simulink model "vehicle_dynamics_system"  (Simulink 7.7)
settings: Solver=ode3  StartTime=0.0  StopTime=10.0  FixedStep=T  RelTol=1e-3
PreLoadFcn:
  | init_parameters;
values from neighbouring files (symbols this model uses):
  CarBody =     [VehicleData_VectorCar.mat]
  Differential =     [VehicleData_VectorCar.mat]
  Engine =     [VehicleData_VectorCar.mat]
  Gearbox =     [VehicleData_VectorCar.mat]
  Ground =     [GroundData_Plane.mat]
  Suspension =     [VehicleData_VectorCar.mat]
  Wheel =     [VehicleData_VectorCar.mat]
libraries: vehicle_dynamics_lib x11, simulink x1
(part 1 of 3)
CloseFcn:
  | rtwprivate ssgencode ModelCloseRequest vehicle_dynamics_system
settings Model: Creator=vismso  LastModifiedBy=visjf
settings DataIOCC: SaveOutput=off  SignalLogging=off  SaveTime=off
settings OptimizationCC: InlineParams=on  UseIntDivNetSlope=on  SimCompilerOptimization=On
settings DebuggingCC: ArtificialAlgebraicLoopMsg=none  BusObjectLabelMismatch=error  RootOutportRequireBusObject=error  StrictBusMsg=Warning
settings SFSimCC: SimParseCustomCode=off
settings RTWCC: SystemTargetFile=cn.tlc  TemplateMakefile=cn_msdll.tmf  Description=Vector CANoe Real-Time Target DLL (Visual C/C++ Project Makefile)  ProcessScript=cn_make_rtw_hook
settings CodeAppCC: MaxIdLength=128  SimulinkBlockComments=off
settings STFCustomTargetCC: FunctionExecutionProfile=off  GeneratePreprocessorConditionals=Disable all  MatFileLogging=on  SystemTargetFile=cn.tlc
settings GRTTargetCC: ParMdlRefBuildCompliant=off  CompOptLevelCompliant=off  ExtModeMexFile=noextcomm  RTWCAPISignals=on  RTWCAPIParams=on
settings CustomProperty: DataType=string  Value=..\canoe

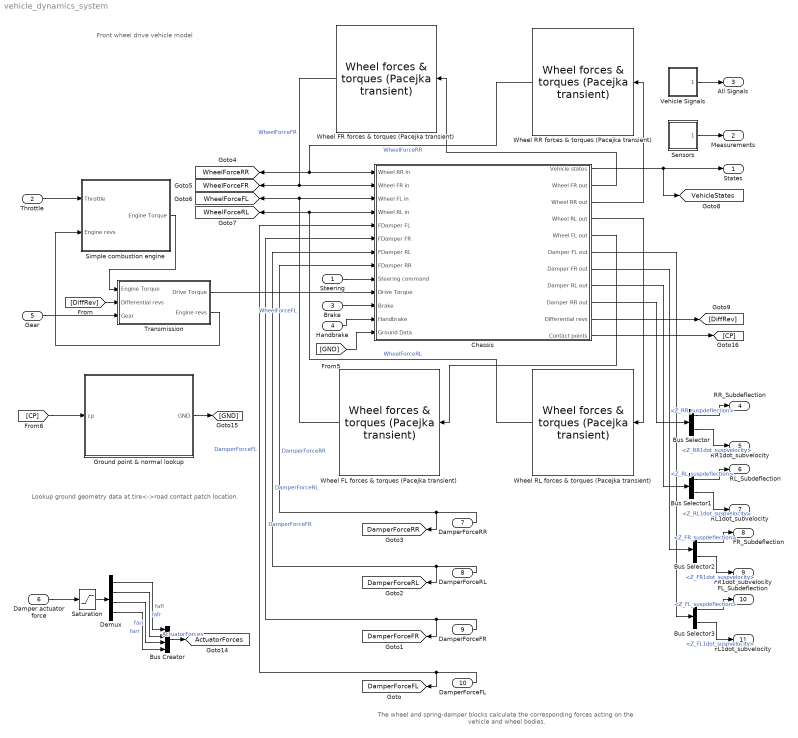
== system vehicle_dynamics_system ==
  note: Front wheel drive vehicle model
  note: The wheel and spring-damper blocks calculate
      | the corresponding forces acting on the vehicle and wheel bodies.
  note: Lookup ground geometry data
      | at tire<->road contact patch location.
  Steering : Inport
  Throttle : Inport  Port=2
  Brake : Inport  Port=3
  Handbrake : Inport  Port=4
  Gear : Inport  Port=5
  Damper actuator force : Inport  Port=6
  "DamperForceRR " : Inport  Port=7
  "DamperForceRL " : Inport  Port=8
  DamperForceFR : Inport  Port=9
  DamperForceFL : Inport  Port=10
  Bus Creator : BusCreator
  Bus Selector : BusSelector  OutputSignals=Z_RR_suspdeflection,Z_RR1dot_suspvelocity
  Bus Selector1 : BusSelector  OutputSignals=Z_RL_suspdeflection,Z_RL1dot_suspvelocity
  Bus Selector2 : BusSelector  OutputSignals=Z_FR_suspdeflection,Z_FR1dot_suspvelocity
  Bus Selector3 : BusSelector  OutputSignals=Z_FL_suspdeflection,Z_FL1dot_suspvelocity
  Chassis : Subsystem  mask{rFLWheelMountPoint=Suspension.MountPointFL, rFRWheelMountPoint=Suspension.MountPointFR, rRLWheelMountPoint=Suspension.MountPointRL, rRRWheelMountPoint=Suspension.MountPointRR, rFAirPointOfAttack=CarBody.FrontAirDragPointOfAttack, rRAirPointOfAttack=CarBody.RearAirDragPointOfAttack, g=9.81, c_ROLLBARF=Suspension.FrontRollbarStiffness, c_ROLLBARR=Suspension.RearRollbarStiffness, m_body=CarBody.Mass, m_wheel=Wheel.Mass, I_body=CarBody.InertiaTensor, I_wheel=Wheel.InertiaTensor}
      mask prompts: rFLWheelMountPoint "Mount point of front left damper in local body coordinates [m]"; rFRWheelMountPoint "Mount point of front right damper in local body coordinates [m]"; rRLWheelMountPoint "Mount point of rear left damper in local body coordinates [m]"; rRRWheelMountPoint "Mount point of rear right damper in local body coordinates [m]"; rFAirPointOfAttack "Front air drag force's point of attack in local body coordinates [m]"; rRAirPointOfAttack "Rear air drag force's point of attack in local body coordinates [m]"; g "Gravity in z-Direction [m/s^2]"; c_ROLLBARF "Front rollbar stiffness [N/m]"; c_ROLLBARR "Rear rollbar stiffness [N/m]"; m_body "Chassis mass [kg]"; m_wheel "Wheel mass [kg]"; I_body "Chassis inertia [kg m^2]"; I_wheel "Wheel inertia [kg m^2]"
      mask init:
      | inputs=find_system(gcb,'SearchDepth',1,'LookUnderMasks','on','BlockType','Inport');
      | outputs=find_system(gcb,'SearchDepth',1,'LookUnderMasks','on','BlockType','Outport');
      | 
      | for i = 1:length(inputs)
      |     s.(['inport' num2str(i)]) = str2num(get_param(inputs{i},'Port'));
      |     s.(['inname' num2str(i)]) = get_param(inputs{i},'Name');
      | end
      | 
      | for i = 1:length(outputs)
      |     s.(['outport' num2str(i)]) = str2num(get_param(outputs{i},'Port'));
      |     s.(['outname' num2str(i)]) = get_param(outputs{i},'Name');
      | end
      settings: MinAlgLoopOccurrences=on
      mask Display:
      | image(imread('chassis.jpg'))
      | 
      | color('white')
      | 
      | port_label('input',s.inport1,s.inname1)
      | port_label('input',s.inport2,s.inname2)
      | port_label('input',s.inport3,s.inname3)
      | port_label('input',s.inport4,s.inname4)
      | port_label('input',s.inport5,s.inname5)
      | port_label('input',s.inport6,s.inname6)
      | port_label('input',s.inport7,s.inname7)
      | port_label('input',s.inport8,s.inname8)
      | port_label('input',s.inport9,s.inname9)
      | port_label('input',s.inport10,s.inname10)
      | port_label('input',s.inport11,s.inname11)
      | port_label('input',s.inport12,s.inname12)
      | port_label('input',s.inport13,s.inname13)
      | 
      | port_label('output',s.outport1,s.outname1)
      | port_label('output',s.outport2,s.outname2)
      | port_label('output',s.outport3,s.outname3)
      | port_label('output',s.outport4,s.outname4)
      | port_label('output',s.outport5,s.outname5)
      | port_label('output',s.outport6,s.outname6)
      | port_label('output',s.outport7,s.outname7)
      | port_label('output',s.outport8,s.outname8)
      | port_label('output',s.outport9,s.outname9)
      | port_label('output',s.outport10,s.outname10)
      | port_label('output',s.outport11,s.outname11)
  Demux : Demux
  Ground point & normal lookup : Subsystem  mask{X=Ground.X, Y=Ground.Y, Z=Ground.Z, Nx=Ground.NormalX, Ny=Ground.NormalY, Nz=Ground.NormalZ}
      mask prompts: X "Ground X grid"; Y "Ground Y grid"; Z "Ground Z values"; Nx "Ground normals (x component)"; Ny "Ground normals (y component)"; Nz "Ground normals (x component)"
      mask Display:
      | image(imread('asphalt.jpg'))
      | color('white')
      | port_label('output',1,'Ground Data')
      | port_label('input',1,'Contact Point')
  Saturation : Saturate  UpperLimit=6e3  LowerLimit=-6e3
  Sensors : Subsystem
      mask init:
      | x=-1:0.05:1;
      | y=sqrt(1-x.^2);
      mask Display:
      | plot((x+1)/2,y/2+.5)
      | plot([0 1/sqrt(2)]/2.5+.5,[0,1/sqrt(2)]/2.5+.5)
  Simple combustion engine : Subsystem
      mask init: same as vehicle_dynamics_system/Chassis
      mask Display:
      | image(imread('engine.jpg'))
      | 
      | color('white')
      | 
      | port_label('input',s.inport1,s.inname1)
      | port_label('input',s.inport2,s.inname2)
      | 
      | port_label('output',s.outport1,s.outname1)
  Transmission : Subsystem  mask(Transmission Block){nGears=Gearbox.Ratios}
      mask prompts: nGears "Gear ratios (1st entry is reverse gear and should be negative)"
      mask help:
      | This block represents the transmission of a vehicle. Set the gear ratios in
      | the input field. Any number of gears greater than zero ist allowed. The
      | first entry usually represents the ratio of the reverse gear and should
      | therefor be negative.
      |
      | Example: [-4;3.827;2.793;2.039;1.488;1.086;0.793]
      | This defines 7 gears.
      mask Help:
      | This block represents the transmission of a vehicle. Set the gear ratios in
      | the input field. Any number of gears greater than zero ist allowed. The
      | first entry usually represents the ratio of the reverse gear and should
      | therefor be negative.
      | 
      | Example: [-4;3.827;2.793;2.039;1.488;1.086;0.793]
      | 
      | This defines 7 gears:
      | R:  -4
      | 1:  3.827
      | 2:  2.793
      | 3:  2.039
      | 4:  1.488
      | 5:  1.086
      | 6:  0.793
      | 
      | With the GEAR input you can select the used gear. A zero at the input means
      | using the first defined ratio, in this case the reverse gear.
      | 
      | The ENGINE REVS output calculates the engine's revs in rad/s according to
      | the DIFFERENTIAL REVS input: omega_engine = GearRatio * omega_diff
      | 
      | The DRIVE TORQUE output calculates the torque applied to the diff with
      | respect to the ENGINE TORQUE input: M_diff = GearRatio * M_engine
  Vehicle Signals : Subsystem
      mask init:
      | x=-1:0.05:1;
      | y=sqrt(1-x.^2);
      mask Display:
      | plot((x+1)/2,y/2+.5)
      | plot([0 1/sqrt(2)]/2.5+.5,[0,1/sqrt(2)]/2.5+.5)
  Wheel FL forces & torques (Pacejka transient) : vehicle_dynamics_lib/Force elements/Wheel forces & torques (Pacejka transient)  SystemSampleTime=-1  c=Wheel.TireStiffness  d=Wheel.TireDamping  r0=Wheel.UnloadedRadius  a=Wheel.PacejkaLateral  b=Wheel.PacejkaLongitudinal  Lx=Wheel.RelaxationLongitudinal  Ly=Wheel.RelaxationLateral  Vlow=Wheel.SlipDampingLowerSpeedLimit
  Wheel FR forces & torques (Pacejka transient) : vehicle_dynamics_lib/Force elements/Wheel forces & torques (Pacejka transient)  SystemSampleTime=-1  c=Wheel.TireStiffness  d=Wheel.TireDamping  r0=Wheel.UnloadedRadius  a=Wheel.PacejkaLateral  b=Wheel.PacejkaLongitudinal  Lx=Wheel.RelaxationLongitudinal  Ly=Wheel.RelaxationLateral  Vlow=Wheel.SlipDampingLowerSpeedLimit
  Wheel RL forces & torques (Pacejka transient) : vehicle_dynamics_lib/Force elements/Wheel forces & torques (Pacejka transient)  SystemSampleTime=-1  c=Wheel.TireStiffness  d=Wheel.TireDamping  r0=Wheel.UnloadedRadius  a=Wheel.PacejkaLateral  b=Wheel.PacejkaLongitudinal  Lx=Wheel.RelaxationLongitudinal  Ly=Wheel.RelaxationLateral  Vlow=Wheel.SlipDampingLowerSpeedLimit
  Wheel RR forces & torques (Pacejka transient) : vehicle_dynamics_lib/Force elements/Wheel forces & torques (Pacejka transient)  SystemSampleTime=-1  c=Wheel.TireStiffness  d=Wheel.TireDamping  r0=Wheel.UnloadedRadius  a=Wheel.PacejkaLateral  b=Wheel.PacejkaLongitudinal  Lx=Wheel.RelaxationLongitudinal  Ly=Wheel.RelaxationLateral  Vlow=Wheel.SlipDampingLowerSpeedLimit
  States : Outport  OutDataTypeStr=Bus: Bus_Vehicle
  Measurements : Outport  Port=2  OutDataTypeStr=Bus: Bus_Measurements
  All Signals : Outport  Port=3  OutDataTypeStr=Bus: Bus_VehicleSignals
  RR_Subdeflection : Outport  Port=4
  RR1dot_subvelocity : Outport  Port=5
  RL_Subdeflection : Outport  Port=6
  RL1dot_subvelocity : Outport  Port=7
  FR_Subdeflection : Outport  Port=8
  FR1dot_subvelocity : Outport  Port=9
  FL_Subdeflection : Outport  Port=10
  FL1dot_subvelocity : Outport  Port=11
  tag scope: ActuatorForces=global, DamperForceFL=global, DamperForceFR=global, DamperForceRL=global, DamperForceRR=global, VehicleStates=global, WheelForceFL=global, WheelForceFR=global, WheelForceRL=global, WheelForceRR=global
  wires:
  Wheel FL forces & torques (Pacejka transient)/1 -> Chassis/3(Wheel FL in), [WheelForceFL]  "WheelForceFL"
  Chassis/5(Wheel FL out) -> Wheel FL forces & torques (Pacejka transient)/1
  Chassis/2(Wheel FR out) -> Wheel FR forces & torques (Pacejka transient)/1
  Wheel FR forces & torques (Pacejka transient)/1 -> Chassis/2(Wheel FR in), [WheelForceFR]  "WheelForceFR"
  Chassis/4(Wheel RL out) -> Wheel RL forces & torques (Pacejka transient)/1
  Chassis/3(Wheel RR out) -> Wheel RR forces & torques (Pacejka transient)/1
  Wheel RR forces & torques (Pacejka transient)/1 -> Chassis/1(Wheel RR in), [WheelForceRR]  "WheelForceRR"
  Wheel RL forces & torques (Pacejka transient)/1 -> Chassis/4(Wheel RL in), [WheelForceRL]  "WheelForceRL"
  Chassis/6(Damper FL out) -> Bus Selector3/1
  Chassis/7(Damper FR out) -> Bus Selector2/1
  Chassis/8(Damper RL out) -> Bus Selector1/1
  Chassis/9(Damper RR out) -> Bus Selector/1
  DamperForceFL/1 -> [DamperForceFL], Chassis/5(FDamper FL)  "DamperForceFL"
  DamperForceFR/1 -> [DamperForceFR], Chassis/6(FDamper FR)  "DamperForceFR"
  "DamperForceRL "/1 -> [DamperForceRL], Chassis/7(FDamper RL)  "DamperForceRL"
  "DamperForceRR "/1 -> [DamperForceRR], Chassis/8(FDamper RR)  "DamperForceRR"
  Chassis/1(Vehicle states) -> States/1, [VehicleStates]
  Steering/1 -> Chassis/9(Steering command)
  Throttle/1 -> Simple combustion engine/1(Throttle)
  Transmission/1(Drive Torque) -> Chassis/10(Drive Torque)
  Simple combustion engine/1(Engine Torque) -> Transmission/1(Engine Torque)
  Transmission/2(Engine revs) -> Simple combustion engine/2(Engine revs)
  Gear/1 -> Transmission/3(Gear)
  Brake/1 -> Chassis/11(Brake)
  Sensors/1(Measurements) -> Measurements/1
  Damper actuator force/1 -> Saturation/1
  [DiffRev] -> Transmission/2(Differential revs)
  Chassis/10(Differential revs) -> [DiffRev]
  Demux/1 -> Bus Creator/1  "fafl"
  Demux/2 -> Bus Creator/2  "fafr"
  Demux/3 -> Bus Creator/3  "farl"
  Demux/4 -> Bus Creator/4  "farr"
  Handbrake/1 -> Chassis/12(Handbrake)
  [GND] -> Chassis/13(Ground Data)
  Ground point & normal lookup/1(GND) -> [GND]
  [CP] -> Ground point & normal lookup/1(cp)
  Chassis/11(Contact points) -> [CP]
  Saturation/1 -> Demux/1
  Bus Creator/1 -> [ActuatorForces]  "ActuatorForces"
  Vehicle Signals/1(Vehicle Signals) -> All Signals/1
  Bus Selector/1 -> RR_Subdeflection/1  "<Z_RR_suspdeflection>"
  Bus Selector/2 -> RR1dot_subvelocity/1  "<Z_RR1dot_suspvelocity>"
  Bus Selector1/1 -> RL_Subdeflection/1  "<Z_RL_suspdeflection>"
  Bus Selector1/2 -> RL1dot_subvelocity/1  "<Z_RL1dot_suspvelocity>"
  Bus Selector2/1 -> FR_Subdeflection/1  "<Z_FR_suspdeflection>"
  Bus Selector2/2 -> FR1dot_subvelocity/1  "<Z_FR1dot_suspvelocity>"
  Bus Selector3/1 -> FL_Subdeflection/1  "<Z_FL_suspdeflection>"
  Bus Selector3/2 -> FL1dot_subvelocity/1  "<Z_FL1dot_suspvelocity>"

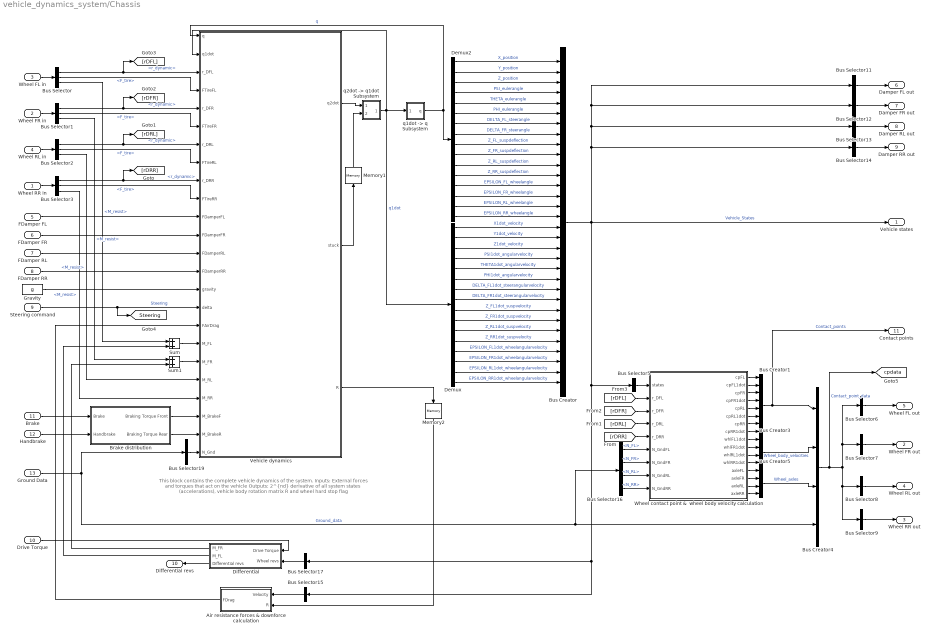
== system vehicle_dynamics_system/Chassis ==
  note: This block contains the complete vehicle dynamics of the system.
      | Inputs: External forces and torques that act on the vehicle
      | Outputs: 2^{nd} derivative of all system states (accelerations), vehicle body rotation matrix R and wheel hard stop flag
  Wheel RR in : Inport
  Wheel FR in : Inport  Port=2
  Wheel FL in : Inport  Port=3
  Wheel RL in : Inport  Port=4
  FDamper FL : Inport  Port=5
  FDamper FR : Inport  Port=6
  FDamper RL : Inport  Port=7
  FDamper RR : Inport  Port=8
  Steering command : Inport  Port=9
  Drive Torque : Inport  Port=10
  Brake : Inport  Port=11
  Handbrake : Inport  Port=12
  Ground Data : Inport  Port=13
  Air resistance forces & downforce calculation : Subsystem  mask{Cw=0.37, Ksfront=0.12, Ksrear=0.16, rho=1.2, A=1.85}
      mask prompts: Cw "Drag coefficient"; Ksfront "Front wing coefficient"; Ksrear "Rear wing coefficient"; rho "Air density [kg/m^3]"; A "Frontal area [m^2]"
  Brake distribution : Subsystem  mask{nBrakeF=0.8, M_Max=4000, M_HBMax=1000}
      mask prompts: nBrakeF "Braking force distribution to front wheels"; M_Max "Maximum braking torque [Nm]"; M_HBMax "Maximum handbrake torque [Nm]"
      mask CallbackString:
      | if or(str2num(get_param(gcb, 'nBrakeF'))<0, str2num(get_param(gcb, 'nBrakeF'))>1)
      | 	error('Brake distribution must be between zero and one.')
      | end||
  Bus Creator : BusCreator  Inputs=32
  Bus Creator1 : BusCreator  Inputs=8
  Bus Creator3 : BusCreator
  Bus Creator4 : BusCreator
  Bus Creator5 : BusCreator
  Bus Selector{,1..3} (4 alike) : BusSelector  OutputSignals=r_dynamic,F_tire,M_resist
  Bus Selector11 : BusSelector  OutputSignals=Z_FL_suspdeflection,Z_FL1dot_suspvelocity  OutputAsBus=on
  Bus Selector12 : BusSelector  OutputSignals=Z_FR_suspdeflection,Z_FR1dot_suspvelocity  OutputAsBus=on
  Bus Selector13 : BusSelector  OutputSignals=Z_RL_suspdeflection,Z_RL1dot_suspvelocity  OutputAsBus=on
  Bus Selector14 : BusSelector  OutputSignals=Z_RR_suspdeflection,Z_RR1dot_suspvelocity  OutputAsBus=on
  Bus Selector15 : BusSelector  OutputSignals=X1dot_velocity,Y1dot_velocity,Z1dot_velocity  OutputAsBus=on
  Bus Selector16 : BusSelector  OutputSignals=GND_FL.N_FL,GND_FR.N_FR,GND_RL.N_RL,GND_RR.N_RR
  Bus Selector17 : BusSelector  OutputSignals=EPSILON_FL1dot_wheelangularvelocity,EPSILON_FR1dot_wheelangularvelocity  OutputAsBus=on
  Bus Selector19 : BusSelector  OutputSignals=GND_FL.N_FL,GND_FR.N_FR,GND_RL.N_RL,GND_RR.N_RR  OutputAsBus=on
  Bus Selector5 : BusSelector  OutputSignals=X_position,Y_position,Z_position,PSI_eulerangle,THETA_eulerangle,PHI_eulerangle,DELTA_FL_steerangle,DELTA_FR_steerangle,Z_FL_suspdeflection,Z_FR_suspdeflection,Z_RL_suspdeflection,Z_RR_suspdeflection,X1dot_velocity,Y1dot_velocity,Z1dot_velocity,PSI1dot_angularvelocity,THETA1dot_angularvelocity,PHI1dot_angularvelocity,Z_FL1dot_suspvelocity,Z_FR1dot_suspvelocity,Z_RL1dot_suspvelocity,Z_RR1dot_suspvelocity,EPSILON_FL1dot_wheelangularvelocity,EPSILON_FR1dot_wheelangularvelocity,EPSILON_RL1dot_wheelangularvelocity,EPSILON_RR1dot_wheelangularvelocity  OutputAsBus=on
  Bus Selector6 : BusSelector  OutputSignals=Wheel_axles.axleFL,Contact_points.cpFL,Contact_points.cpFL1dot,Wheel_body_velocities.whlFL1dot,Ground_data.GND_FL  OutputAsBus=on
  Bus Selector7 : BusSelector  OutputSignals=Wheel_axles.axleFR,Contact_points.cpFR,Contact_points.cpFR1dot,Wheel_body_velocities.whlFR1dot,Ground_data.GND_FR  OutputAsBus=on
  Bus Selector8 : BusSelector  OutputSignals=Wheel_axles.axleRL,Contact_points.cpRL,Contact_points.cpRL1dot,Wheel_body_velocities.whlRL1dot,Ground_data.GND_RL  OutputAsBus=on
  Bus Selector9 : BusSelector  OutputSignals=Wheel_axles.axleRR,Contact_points.cpRR,Contact_points.cpRR1dot,Wheel_body_velocities.whlRR1dot,Ground_data.GND_RR  OutputAsBus=on
  Demux : Demux  Outputs=16
  Demux2 : Demux  Outputs=16
  Differential : Subsystem  mask{nd=Differential.Ratio}
      mask prompts: nd "Differential ratio"
  Gravity : Constant  Value=g
  Memory1 : Memory
  Memory2 : Memory
  Sum : Sum
  Sum1 : Sum
  Vehicle dynamics : Stateflow chart  RequirementInfo={} %GIDa_b7f5b320_cde6_4ae1_9d3b_3c9937b9ba5b  TreatAsAtomicUnit=on
  Wheel contact point &  wheel body velocity calculation : Stateflow chart  TreatAsAtomicUnit=on
      settings: MinAlgLoopOccurrences=on
  "q1dot -> q Subsystem" : Subsystem
      mask Display:
      | droots([],[0],1)
      | plot([1 1.5 1.7 2],[0 0 2 2])
      | plot(6,6)
  "q2dot -> q1dot Subsystem" : Subsystem
      mask Display:
      | droots([],[0],1)
      | plot([1 1 2 2],[0 2 2 0])
      | plot([2 2.4 2.4],[2 2 0])
      | plot(7,7)
  Vehicle states : Outport
  Wheel FR out : Outport  Port=2
  Wheel RR out : Outport  Port=3
  Wheel RL out : Outport  Port=4
  Wheel FL out : Outport  Port=5
  Damper FL out : Outport  Port=6
  Damper FR out : Outport  Port=7
  Damper RL out : Outport  Port=8
  Damper RR out : Outport  Port=9
  Differential revs : Outport  Port=10
  Contact points : Outport  Port=11
  tag scope: Steering=global, cpdata=global
  wires:
  Vehicle dynamics/1(q2dot) -> "q2dot -> q1dot Subsystem"/1(q2dot)
  "q1dot -> q Subsystem"/1(q) -> Demux2/1, Vehicle dynamics/1(q)  "q"
  Wheel FL in/1 -> Bus Selector/1
  Bus Selector/1 -> Vehicle dynamics/3(r_DFL), [rDFL]  "<r_dynamic>"
  Wheel FR in/1 -> Bus Selector1/1
  Wheel RL in/1 -> Bus Selector2/1
  Wheel RR in/1 -> Bus Selector3/1
  Bus Selector1/1 -> Vehicle dynamics/5(r_DFR), [rDFR]  "<r_dynamic>"
  Bus Selector1/2 -> Vehicle dynamics/6(FTireFR)  "<F_tire>"
  Bus Selector2/1 -> Vehicle dynamics/7(r_DRL), [rDRL]  "<r_dynamic>"
  Bus Selector2/2 -> Vehicle dynamics/8(FTireRL)  "<F_tire>"
  Bus Selector3/1 -> Vehicle dynamics/9(r_DRR), [rDRR]  "<r_dynamic>"
  Bus Selector3/2 -> Vehicle dynamics/10(FTireRR)  "<F_tire>"
  FDamper FL/1 -> Vehicle dynamics/11(FDamperFL)
  FDamper FR/1 -> Vehicle dynamics/12(FDamperFR)
  FDamper RL/1 -> Vehicle dynamics/13(FDamperRL)
  FDamper RR/1 -> Vehicle dynamics/14(FDamperRR)
  Gravity/1 -> Vehicle dynamics/15(gravity)
  Bus Creator/1 -> Vehicle states/1, Bus Selector11/1, Bus Selector12/1, Bus Selector13/1, Bus Selector14/1, Bus Selector5/1, Bus Selector15/1, Bus Selector17/1  "Vehicle_States"
  Demux/1 -> Bus Creator/17  "X1dot_velocity"
  Demux/2 -> Bus Creator/18  "Y1dot_velocity"
  Demux/3 -> Bus Creator/19  "Z1dot_velocity"
  Demux/4 -> Bus Creator/20  "PSI1dot_angularvelocity"
  Demux/5 -> Bus Creator/21  "THETA1dot_angularvelocity"
  Demux/6 -> Bus Creator/22  "PHI1dot_angularvelocity"
  Demux/7 -> Bus Creator/23  "DELTA_FL1dot_steerangularvelocity"
  Demux/8 -> Bus Creator/24  "DELTA_FR1dot_steerangularvelocity"
  Demux/9 -> Bus Creator/25  "Z_FL1dot_suspvelocity"
  Demux/10 -> Bus Creator/26  "Z_FR1dot_suspvelocity"
  Demux/11 -> Bus Creator/27  "Z_RL1dot_suspvelocity"
  Demux/12 -> Bus Creator/28  "Z_RR1dot_suspvelocity"
  Demux/13 -> Bus Creator/29  "EPSILON_FL1dot_wheelangularvelocity"
  Demux/14 -> Bus Creator/30  "EPSILON_FR1dot_wheelangularvelocity"
  Demux/15 -> Bus Creator/31  "EPSILON_RL1dot_wheelangularvelocity"
  Demux/16 -> Bus Creator/32  "EPSILON_RR1dot_wheelangularvelocity"
  Demux2/1 -> Bus Creator/1  "X_position"
  Demux2/2 -> Bus Creator/2  "Y_position"
  Demux2/3 -> Bus Creator/3  "Z_position"
  Demux2/4 -> Bus Creator/4  "PSI_eulerangle"
  Demux2/5 -> Bus Creator/5  "THETA_eulerangle"
  Demux2/6 -> Bus Creator/6  "PHI_eulerangle"
  Demux2/9 -> Bus Creator/9  "Z_FL_suspdeflection"
  Demux2/10 -> Bus Creator/10  "Z_FR_suspdeflection"
  Demux2/11 -> Bus Creator/11  "Z_RL_suspdeflection"
  Demux2/12 -> Bus Creator/12  "Z_RR_suspdeflection"
  Demux2/13 -> Bus Creator/13  "EPSILON_FL_wheelangle"
  Demux2/14 -> Bus Creator/14  "EPSILON_FR_wheelangle"
  Demux2/15 -> Bus Creator/15  "EPSILON_RL_wheelangle"
  Demux2/16 -> Bus Creator/16  "EPSILON_RR_wheelangle"
  Steering command/1 -> Vehicle dynamics/16(delta), [Steering]  "Steering"
  Demux2/7 -> Bus Creator/7  "DELTA_FL_steerangle"
  Demux2/8 -> Bus Creator/8  "DELTA_FR_steerangle"
  Bus Creator1/1 -> Bus Creator4/1, Contact points/1  "Contact_points"
  Wheel contact point &  wheel body velocity calculation/1(cpFL) -> Bus Creator1/1
  Wheel contact point &  wheel body velocity calculation/2(cpFL1dot) -> Bus Creator1/2
  Wheel contact point &  wheel body velocity calculation/3(cpFR) -> Bus Creator1/3
  Wheel contact point &  wheel body velocity calculation/4(cpFR1dot) -> Bus Creator1/4
  Wheel contact point &  wheel body velocity calculation/5(cpRL) -> Bus Creator1/5
  Wheel contact point &  wheel body velocity calculation/6(cpRL1dot) -> Bus Creator1/6
  Wheel contact point &  wheel body velocity calculation/7(cpRR) -> Bus Creator1/7
  Wheel contact point &  wheel body velocity calculation/8(cpRR1dot) -> Bus Creator1/8
  Wheel contact point &  wheel body velocity calculation/9(whlFL1dot) -> Bus Creator3/1
  Wheel contact point &  wheel body velocity calculation/10(whlFR1dot) -> Bus Creator3/2
  Wheel contact point &  wheel body velocity calculation/11(whlRL1dot) -> Bus Creator3/3
  Wheel contact point &  wheel body velocity calculation/12(whlRR1dot) -> Bus Creator3/4
  Bus Selector5/1 -> Wheel contact point &  wheel body velocity calculation/1(states)
  Bus Creator4/1 -> Bus Selector7/1, Bus Selector6/1, Bus Selector9/1, Bus Selector8/1, [cpdata]  "Contact_point_data"
  Bus Selector6/1 -> Wheel FL out/1
  Bus Selector7/1 -> Wheel FR out/1
  Bus Selector8/1 -> Wheel RL out/1
  Bus Selector9/1 -> Wheel RR out/1
  Bus Selector11/1 -> Damper FL out/1
  Bus Selector12/1 -> Damper FR out/1
  Bus Selector13/1 -> Damper RL out/1
  Bus Selector14/1 -> Damper RR out/1
  Bus Selector15/1 -> Air resistance forces & downforce calculation/1(Velocity)
  Air resistance forces & downforce calculation/1(FDrag) -> Vehicle dynamics/17(FAirDrag)
  Sum/1 -> Vehicle dynamics/18(M_FL)
  Sum1/1 -> Vehicle dynamics/19(M_FR)
  Bus Selector/3 -> Sum/1  "<M_resist>"
  Bus Selector1/3 -> Sum1/1  "<M_resist>"
  Bus Selector2/3 -> Vehicle dynamics/20(M_RL)  "<M_resist>"
  Bus Selector3/3 -> Vehicle dynamics/21(M_RR)  "<M_resist>"
  Bus Creator5/1 -> Bus Creator4/3  "Wheel_axles"
  Wheel contact point &  wheel body velocity calculation/13(axleFL) -> Bus Creator5/1
  Wheel contact point &  wheel body velocity calculation/14(axleFR) -> Bus Creator5/2
  Wheel contact point &  wheel body velocity calculation/15(axleRL) -> Bus Creator5/3
  Wheel contact point &  wheel body velocity calculation/16(axleRR) -> Bus Creator5/4
  Bus Creator3/1 -> Bus Creator4/2  "Wheel_body_velocities"
  Drive Torque/1 -> Differential/1(Drive Torque)
  Differential/2(M_FL) -> Sum/2
  Differential/1(M_FR) -> Sum1/2
  Bus Selector17/1 -> Differential/2(Wheel revs)
  Differential/3(Differential revs) -> Differential revs/1
  [rDFL] -> Wheel contact point &  wheel body velocity calculation/2(r_DFL)
  [rDFR] -> Wheel contact point &  wheel body velocity calculation/3(r_DFR)
  [rDRL] -> Wheel contact point &  wheel body velocity calculation/4(r_DRL)
  [rDRR] -> Wheel contact point &  wheel body velocity calculation/5(r_DRR)
  Brake/1 -> Brake distribution/1(Brake)
  Brake distribution/1(Braking Torque Front) -> Vehicle dynamics/22(M_BrakeF)
  Brake distribution/2(Braking Torque Rear) -> Vehicle dynamics/23(M_BrakeR)
  Vehicle dynamics/3(R) -> Memory2/1
  "q2dot -> q1dot Subsystem"/1(q1dot) -> Demux/1, Vehicle dynamics/2(q1dot), "q1dot -> q Subsystem"/1(q1dot)  "q1dot"
  Vehicle dynamics/2(stuck) -> Memory1/1
  Memory2/1 -> Air resistance forces & downforce calculation/2(R)
  Memory1/1 -> "q2dot -> q1dot Subsystem"/2(Wheel revs reset)
  Ground Data/1 -> Bus Selector19/1, Bus Selector16/1, Bus Creator4/4  "Ground_data"
  Bus Selector16/1 -> Wheel contact point &  wheel body velocity calculation/6(N_GndFL)  "<N_FL>"
  Bus Selector16/2 -> Wheel contact point &  wheel body velocity calculation/7(N_GndFR)  "<N_FR>"
  Bus Selector16/3 -> Wheel contact point &  wheel body velocity calculation/8(N_GndRL)  "<N_RL>"
  Bus Selector16/4 -> Wheel contact point &  wheel body velocity calculation/9(N_GndRR)  "<N_RR>"
  Bus Selector19/1 -> Vehicle dynamics/24(N_Gnd)
  Handbrake/1 -> Brake distribution/2(Handbrake)
  Bus Selector/2 -> Vehicle dynamics/4(FTireFL)  "<F_tire>"

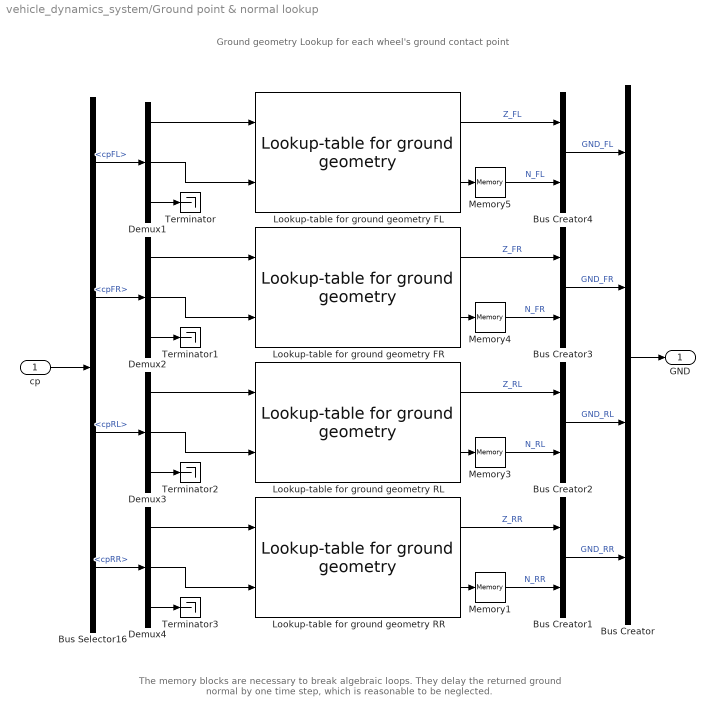
== system vehicle_dynamics_system/Ground point & normal lookup ==
  note: The memory blocks are necessary to break algebraic loops.
      | They delay the returned ground normal by one time step, which
      | is reasonable to be neglected.
  note: Ground geometry Lookup for each wheel's ground contact point
  cp : Inport
  Bus Creator : BusCreator
  Bus Creator{1..4} (4 alike) : BusCreator  Inputs=2
  Bus Selector16 : BusSelector  OutputSignals=cpFL,cpFR,cpRL,cpRR
  Demux{1..4} (4 alike) : Demux  Outputs=3
  Lookup-table for ground geometry FL : vehicle_dynamics_lib/Helper blocks/Lookup-table for ground geometry  SystemSampleTime=-1
  Lookup-table for ground geometry FR : vehicle_dynamics_lib/Helper blocks/Lookup-table for ground geometry  SystemSampleTime=-1
  Lookup-table for ground geometry RL : vehicle_dynamics_lib/Helper blocks/Lookup-table for ground geometry  SystemSampleTime=-1
  Lookup-table for ground geometry RR : vehicle_dynamics_lib/Helper blocks/Lookup-table for ground geometry  SystemSampleTime=-1
  Memory{1,3..5} (4 alike) : Memory  X0=[0;0;1]
  Terminator{,1..3} (4 alike) : Terminator
  GND : Outport
  wires:
  Bus Selector16/1 -> Demux1/1  "<cpFL>"
  cp/1 -> Bus Selector16/1
  Bus Selector16/2 -> Demux2/1  "<cpFR>"
  Bus Selector16/3 -> Demux3/1  "<cpRL>"
  Bus Selector16/4 -> Demux4/1  "<cpRR>"
  Demux1/1 -> Lookup-table for ground geometry FL/1
  Demux1/2 -> Lookup-table for ground geometry FL/2
  Demux2/1 -> Lookup-table for ground geometry FR/1
  Demux2/2 -> Lookup-table for ground geometry FR/2
  Demux3/1 -> Lookup-table for ground geometry RL/1
  Demux3/2 -> Lookup-table for ground geometry RL/2
  Demux4/1 -> Lookup-table for ground geometry RR/1
  Demux4/2 -> Lookup-table for ground geometry RR/2
  Demux1/3 -> Terminator/1
  Demux2/3 -> Terminator1/1
  Demux3/3 -> Terminator2/1
  Demux4/3 -> Terminator3/1
  Lookup-table for ground geometry FL/1 -> Bus Creator4/1  "Z_FL"
  Lookup-table for ground geometry FL/2 -> Memory5/1
  Lookup-table for ground geometry FR/1 -> Bus Creator3/1  "Z_FR"
  Lookup-table for ground geometry FR/2 -> Memory4/1
  Lookup-table for ground geometry RL/1 -> Bus Creator2/1  "Z_RL"
  Lookup-table for ground geometry RL/2 -> Memory3/1
  Lookup-table for ground geometry RR/1 -> Bus Creator1/1  "Z_RR"
  Lookup-table for ground geometry RR/2 -> Memory1/1
  Bus Creator4/1 -> Bus Creator/1  "GND_FL"
  Bus Creator3/1 -> Bus Creator/2  "GND_FR"
  Bus Creator2/1 -> Bus Creator/3  "GND_RL"
  Bus Creator1/1 -> Bus Creator/4  "GND_RR"
  Bus Creator/1 -> GND/1
  Memory1/1 -> Bus Creator1/2  "N_RR"
  Memory3/1 -> Bus Creator2/2  "N_RL"
  Memory4/1 -> Bus Creator3/2  "N_FR"
  Memory5/1 -> Bus Creator4/2  "N_FL"

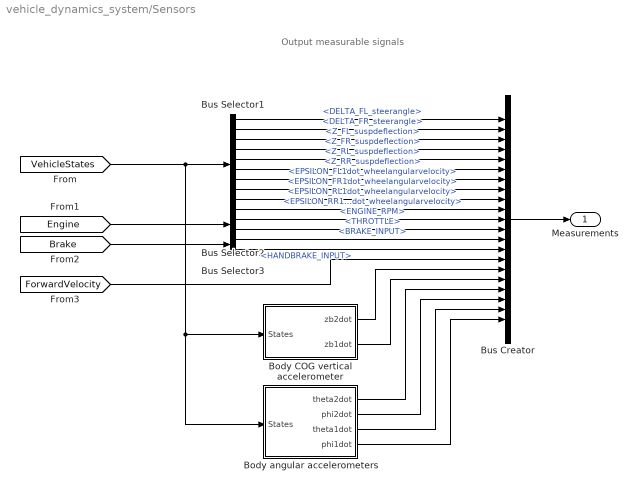
== system vehicle_dynamics_system/Sensors ==
  note: Output measurable signals
  Body COG vertical accelerometer : Subsystem
  Body angular accelerometers : Subsystem
  Bus Creator : BusCreator  Inputs=21
  Bus Selector1 : BusSelector  OutputSignals=DELTA_FL_steerangle,DELTA_FR_steerangle,Z_FL_suspdeflection,Z_FR_suspdeflection,Z_RL_suspdeflection,Z_RR_suspdeflection,EPSILON_FL1dot_wheelangularvelocity,EPSILON_FR1dot_wheelangularvelocity,EPSILON_RL1dot_wheelangularvelocity,EPSILON_RR1dot_wheelangularvelocity
  Bus Selector2 : BusSelector  OutputSignals=ENGINE_RPM,THROTTLE
  Bus Selector3 : BusSelector  OutputSignals=BRAKE_INPUT,HANDBRAKE_INPUT
  Measurements : Outport  OutDataTypeStr=Bus: Bus_Measurements
  wires:
  [VehicleStates] -> Body COG vertical accelerometer/1(States), Body angular accelerometers/1(States), Bus Selector1/1
  [Engine] -> Bus Selector2/1
  [Brake] -> Bus Selector3/1
  Bus Creator/1 -> Measurements/1
  Bus Selector1/1 -> Bus Creator/1  "<DELTA_FL_steerangle>"
  Bus Selector1/2 -> Bus Creator/2  "<DELTA_FR_steerangle>"
  Bus Selector1/3 -> Bus Creator/3  "<Z_FL_suspdeflection>"
  Bus Selector1/4 -> Bus Creator/4  "<Z_FR_suspdeflection>"
  Bus Selector1/5 -> Bus Creator/5  "<Z_RL_suspdeflection>"
  Bus Selector1/6 -> Bus Creator/6  "<Z_RR_suspdeflection>"
  Bus Selector1/7 -> Bus Creator/7  "<EPSILON_FL1dot_wheelangularvelocity>"
  Bus Selector1/8 -> Bus Creator/8  "<EPSILON_FR1dot_wheelangularvelocity>"
  Bus Selector1/9 -> Bus Creator/9  "<EPSILON_RL1dot_wheelangularvelocity>"
  Bus Selector1/10 -> Bus Creator/10  "<EPSILON_RR1dot_wheelangularvelocity>"
  Bus Selector2/1 -> Bus Creator/11  "<ENGINE_RPM>"
  Bus Selector2/2 -> Bus Creator/12  "<THROTTLE>"
  Bus Selector3/1 -> Bus Creator/13  "<BRAKE_INPUT>"
  Bus Selector3/2 -> Bus Creator/14  "<HANDBRAKE_INPUT>"
  [ForwardVelocity] -> Bus Creator/15
  Body COG vertical accelerometer/1(zb2dot) -> Bus Creator/16
  Body COG vertical accelerometer/2(zb1dot) -> Bus Creator/17
  Body angular accelerometers/1(theta2dot) -> Bus Creator/18
  Body angular accelerometers/2(phi2dot) -> Bus Creator/19
  Body angular accelerometers/3(theta1dot) -> Bus Creator/20
  Body angular accelerometers/4(phi1dot) -> Bus Creator/21

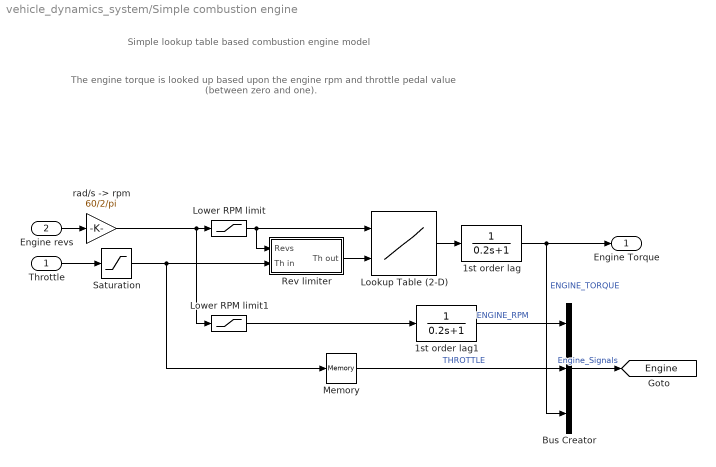
== system vehicle_dynamics_system/Simple combustion engine ==
  note: The engine torque is looked up based upon the engine rpm
      | and throttle pedal value (between zero and one).
  note: Simple lookup table based combustion engine model
  Throttle : Inport  PortDimensions=1
  Engine revs : Inport  Port=2  OutDataTypeStr=double
  1st order lag : TransferFcn  Denominator=[0.2 1]
  1st order lag1 : TransferFcn  Denominator=[0.2 1]
  Bus Creator : BusCreator  Inputs=3
  Lookup Table (2-D) : Lookup2D  RowIndex=Engine.RPM  ColumnIndex=Engine.Throttle  Table=Engine.Torque  OutDataTypeStr=double
  Lower RPM limit : Saturate  UpperLimit=inf  LowerLimit=0
  Lower RPM limit1 : Saturate  UpperLimit=inf  LowerLimit=400
  Memory : Memory
  Rev limiter : Subsystem
  Saturation : Saturate  UpperLimit=1  LowerLimit=0
  "rad/s -> rpm" : Gain  Gain=60/2/pi
  Engine Torque : Outport
  tag scope: Engine=global
  wires:
  Engine revs/1 -> "rad/s -> rpm"/1
  Throttle/1 -> Saturation/1
  Saturation/1 -> Rev limiter/2(Th in), Memory/1
  "rad/s -> rpm"/1 -> Lower RPM limit1/1, Lower RPM limit/1
  Bus Creator/1 -> [Engine]  "Engine_Signals"
  Lower RPM limit1/1 -> 1st order lag1/1
  Lookup Table (2-D)/1 -> 1st order lag/1
  Lower RPM limit/1 -> Lookup Table (2-D)/1, Rev limiter/1(Revs)
  1st order lag/1 -> Engine Torque/1, Bus Creator/3  "ENGINE_TORQUE"
  1st order lag1/1 -> Bus Creator/1  "ENGINE_RPM"
  Rev limiter/1(Th out) -> Lookup Table (2-D)/2
  Memory/1 -> Bus Creator/2  "THROTTLE"

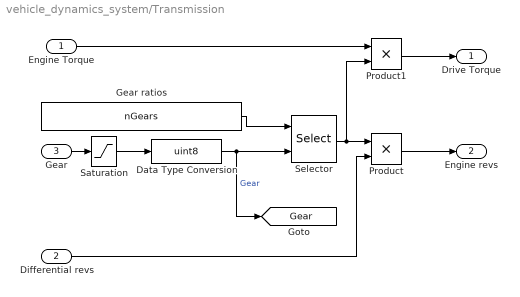
== system vehicle_dynamics_system/Transmission ==
  Engine Torque : Inport
  Differential revs : Inport  Port=2
  Gear : Inport  Port=3
  Data Type Conversion : DataTypeConversion  OutDataTypeStr=uint8  RndMeth=Round  SaturateOnIntegerOverflow=on
  Gear ratios : Constant  Value=nGears
  Product : Product  RndMeth=Zero
  Product1 : Product  RndMeth=Zero
  Saturation : Saturate  UpperLimit=length(nGears)-1  LowerLimit=0
  Selector : Selector  IndexMode=Zero-based  InputPortWidth=7  IndexOptions=Index vector (port)  Indices=[1 3]  OutputSizes=1
  Drive Torque : Outport
  Engine revs : Outport  Port=2
  tag scope: Gear=global
  wires:
  Gear/1 -> Saturation/1
  Data Type Conversion/1 -> Selector/2, [Gear]  "Gear"
  Gear ratios/1 -> Selector/1
  Product/1 -> Engine revs/1
  Selector/1 -> Product/1, Product1/2
  Differential revs/1 -> Product/2
  Engine Torque/1 -> Product1/1
  Product1/1 -> Drive Torque/1
  Saturation/1 -> Data Type Conversion/1

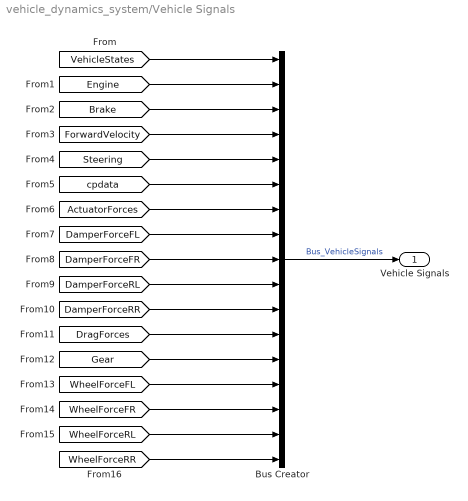
== system vehicle_dynamics_system/Vehicle Signals ==
  Bus Creator : BusCreator  Inputs=17
  Vehicle Signals : Outport  OutDataTypeStr=Bus: Bus_VehicleSignals
  wires:
  [VehicleStates] -> Bus Creator/1
  [Engine] -> Bus Creator/2
  [Brake] -> Bus Creator/3
  [ForwardVelocity] -> Bus Creator/4
  [Steering] -> Bus Creator/5
  [cpdata] -> Bus Creator/6
  [ActuatorForces] -> Bus Creator/7
  [DamperForceFL] -> Bus Creator/8
  [DamperForceFR] -> Bus Creator/9
  [DamperForceRL] -> Bus Creator/10
  [DamperForceRR] -> Bus Creator/11
  [DragForces] -> Bus Creator/12
  [Gear] -> Bus Creator/13
  [WheelForceFL] -> Bus Creator/14
  [WheelForceFR] -> Bus Creator/15
  [WheelForceRL] -> Bus Creator/16
  [WheelForceRR] -> Bus Creator/17
  Bus Creator/1 -> Vehicle Signals/1  "Bus_VehicleSignals"

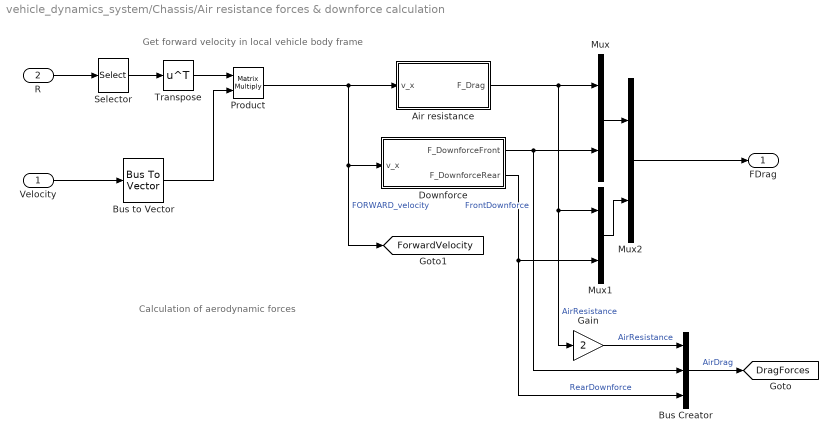
== system vehicle_dynamics_system/Chassis/Air resistance forces & downforce calculation ==
  note: Calculation of aerodynamic forces
  note: Get forward velocity in
      | local vehicle body frame
  Velocity : Inport
  R : Inport  Port=2
  Air resistance : Subsystem
  Bus Creator : BusCreator  Inputs=3
  Bus to Vector : BusToVector
  Downforce : Subsystem
  Gain : Gain  Gain=2
  Mux : Mux  Inputs=2
  Mux1 : Mux  Inputs=2
  Mux2 : Mux  Inputs=2
  Product : Product  Multiplication=Matrix(*)  RndMeth=Zero
  Selector : Selector  NumberOfDimensions=2  InputPortWidth=3  IndexOptions=Index vector (dialog),Index vector (dialog)  Indices=[1:3],[1]  OutputSizes=1,1
  Transpose : Math  Operator=transpose  SaturateOnIntegerOverflow=on
  FDrag : Outport
  tag scope: DragForces=global, ForwardVelocity=global
  wires:
  Velocity/1 -> Bus to Vector/1
  R/1 -> Selector/1
  Transpose/1 -> Product/1
  Bus to Vector/1 -> Product/2
  Selector/1 -> Transpose/1
  Product/1 -> Air resistance/1(v_x), Downforce/1(v_x), [ForwardVelocity]  "FORWARD_velocity"
  Air resistance/1(F_Drag) -> Mux/1, Mux1/1, Gain/1  "AirResistance"
  Downforce/1(F_DownforceFront) -> Mux/2, Bus Creator/2  "FrontDownforce"
  Mux2/1 -> FDrag/1
  Mux/1 -> Mux2/1
  Mux1/1 -> Mux2/2
  Downforce/2(F_DownforceRear) -> Mux1/2, Bus Creator/3  "RearDownforce"
  Bus Creator/1 -> [DragForces]  "AirDrag"
  Gain/1 -> Bus Creator/1  "AirResistance"

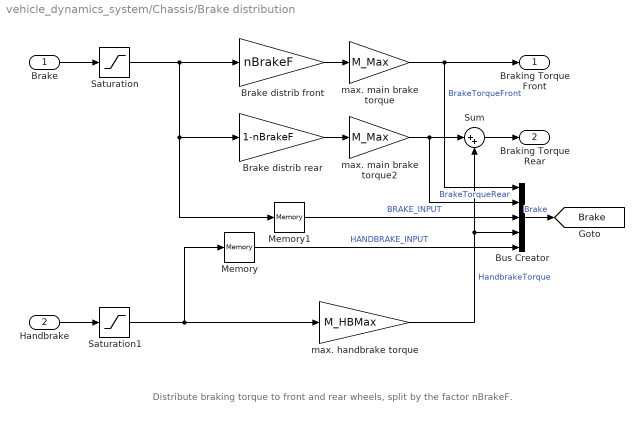
== system vehicle_dynamics_system/Chassis/Brake distribution ==
  note: Distribute braking torque to front and rear wheels, split by the factor nBrakeF.
  Brake : Inport
  Handbrake : Inport  Port=2
  Brake distrib front : Gain  Gain=nBrakeF
  Brake distrib rear : Gain  Gain=1-nBrakeF
  Bus Creator : BusCreator  Inputs=5
  Memory : Memory
  Memory1 : Memory
  Saturation : Saturate  UpperLimit=1  LowerLimit=0
  Saturation1 : Saturate  UpperLimit=1  LowerLimit=0
  Sum : Sum  Inputs=|++
  max. handbrake torque : Gain  Gain=M_HBMax
  max. main brake torque : Gain  Gain=M_Max
  max. main brake torque2 : Gain  Gain=M_Max
  Braking Torque Front : Outport
  Braking Torque Rear : Outport  Port=2
  tag scope: Brake=global
  wires:
  Brake/1 -> Saturation/1
  Brake distrib front/1 -> max. main brake torque/1
  max. main brake torque/1 -> Braking Torque Front/1, Bus Creator/1  "BrakeTorqueFront"
  Brake distrib rear/1 -> max. main brake torque2/1
  max. main brake torque2/1 -> Bus Creator/2, Sum/1  "BrakeTorqueRear"
  Bus Creator/1 -> [Brake]  "Brake"
  Saturation/1 -> Brake distrib front/1, Brake distrib rear/1, Memory1/1
  Handbrake/1 -> Saturation1/1
  Sum/1 -> Braking Torque Rear/1
  Saturation1/1 -> max. handbrake torque/1, Memory/1
  max. handbrake torque/1 -> Sum/2, Bus Creator/4  "HandbrakeTorque"
  Memory/1 -> Bus Creator/5  "HANDBRAKE_INPUT"
  Memory1/1 -> Bus Creator/3  "BRAKE_INPUT"

== system vehicle_dynamics_system/Chassis/Differential ==
  note: Differential (simple)
  note: This is only a simplified model of a diff because
      | the output energy doesn't equal the input energy, i.e.
  note: M_{in} \cdot \omega_{in} \neq M_{FL} \cdot \omega_{FL} + M_{FR} \cdot \omega_{FR}
  Drive Torque : Inport
  Wheel revs : Inport  Port=2
  Bus Selector : BusSelector  OutputSignals=EPSILON_FL1dot_wheelangularvelocity,EPSILON_FR1dot_wheelangularvelocity
  Diff ratio : Gain  Gain=nd
  Diff ratio2 : Gain  Gain=nd
  Gain : Gain  Gain=.5
  Gain2 : Gain  Gain=.5
  Sum : Sum
  M_FR : Outport
  M_FL : Outport  Port=2
  Differential revs : Outport  Port=3
  wires:
  Drive Torque/1 -> Diff ratio/1
  Diff ratio/1 -> Gain/1
  Wheel revs/1 -> Bus Selector/1
  Gain/1 -> M_FL/1, M_FR/1
  Diff ratio2/1 -> Gain2/1
  Gain2/1 -> Differential revs/1
  Sum/1 -> Diff ratio2/1
  Bus Selector/1 -> Sum/1  "<EPSILON_FL1dot_wheelangularvelocity>"
  Bus Selector/2 -> Sum/2  "<EPSILON_FR1dot_wheelangularvelocity>"

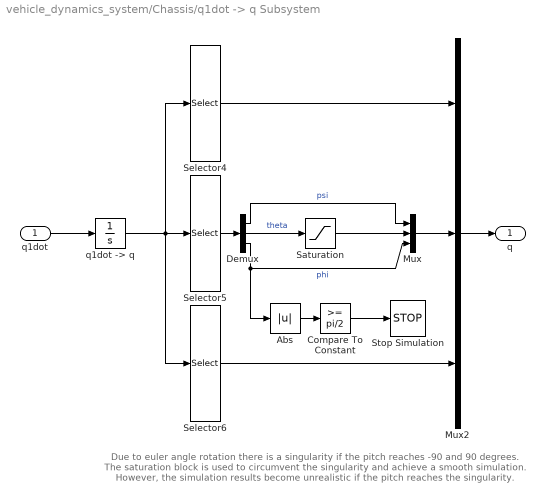
== system vehicle_dynamics_system/Chassis/q1dot -> q Subsystem ==
  note: Due to euler angle rotation there is a singularity if the pitch reaches -90 and 90 degrees.
      | The saturation block is used to circumvent the singularity and achieve a smooth simulation.
      | However, the simulation results become unrealistic if the pitch reaches the singularity.
  q1dot : Inport
  Abs : Abs
  Compare To Constant : simulink/Logic and Bit Operations/Compare To Constant  SystemSampleTime=-1  relop=>=  const=pi/2  LogicOutDataTypeMode=boolean
  Demux : Demux  Outputs=3
  Mux : Mux  Inputs=3
  Mux2 : Mux  Inputs=3
  Saturation : Saturate  UpperLimit=pi/2-0.02  LowerLimit=-pi/2+0.02
  Selector4 : Selector  InputPortWidth=16  IndexOptions=Index vector (dialog)  Indices=[1:3]  OutputSizes=1
  Selector5 : Selector  InputPortWidth=16  IndexOptions=Index vector (dialog)  Indices=[4:6]  OutputSizes=1
  Selector6 : Selector  InputPortWidth=16  IndexOptions=Index vector (dialog)  Indices=[7:16]  OutputSizes=1
  Stop Simulation : Stop
  "q1dot -> q" : Integrator  InitialCondition=[-15;0;0.610;0;3/180*pi;0;0;0;-Suspension.SpringFreeLengthFL;-Suspension.SpringFreeLengthFR;-Suspension.SpringFreeLengthRL;-Suspension.SpringFreeLengthRR;zeros(4,1)]
  q : Outport
  wires:
  q1dot/1 -> "q1dot -> q"/1
  Mux2/1 -> q/1
  Selector4/1 -> Mux2/1
  Mux/1 -> Mux2/2
  Selector6/1 -> Mux2/3
  "q1dot -> q"/1 -> Selector4/1, Selector5/1, Selector6/1
  Selector5/1 -> Demux/1
  Demux/1 -> Mux/1  "psi"
  Demux/3 -> Mux/3, Abs/1  "phi"
  Demux/2 -> Saturation/1  "theta"
  Saturation/1 -> Mux/2
  Abs/1 -> Compare To Constant/1
  Compare To Constant/1 -> Stop Simulation/1

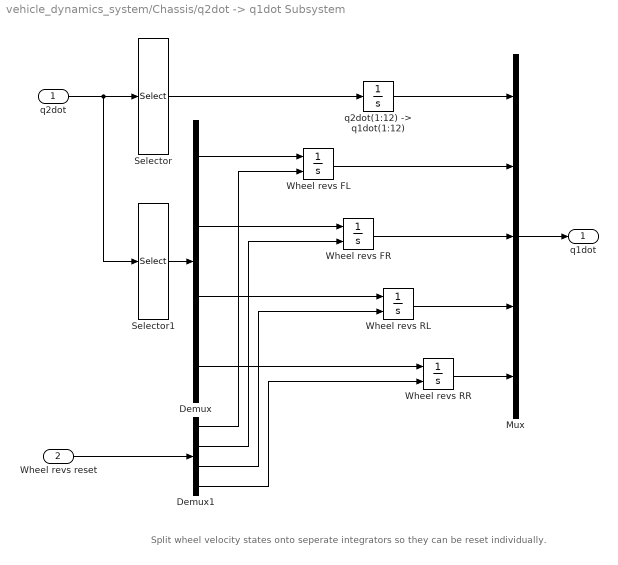
== system vehicle_dynamics_system/Chassis/q2dot -> q1dot Subsystem ==
  note: Split wheel velocity states onto seperate integrators so they can be reset individually.
  q2dot : Inport
  Wheel revs reset : Inport  Port=2  PortDimensions=4
  Demux : Demux
  Demux1 : Demux
  Mux : Mux  Inputs=5
  Selector : Selector  InputPortWidth=16  IndexOptions=Index vector (dialog)  Indices=[1:12]  OutputSizes=1
  Selector1 : Selector  InputPortWidth=16  IndexOptions=Index vector (dialog)  Indices=[13:16]  OutputSizes=1
  Wheel revs FL : Integrator  ExternalReset=level hold
  Wheel revs FR : Integrator  ExternalReset=level hold
  Wheel revs RL : Integrator  ExternalReset=level hold
  Wheel revs RR : Integrator  ExternalReset=level hold
  "q2dot(1:12) -> q1dot(1:12)" : Integrator  InitialCondition=[0;0;0;0;0;0;zeros(6,1)]
  q1dot : Outport
  wires:
  Mux/1 -> q1dot/1
  "q2dot(1:12) -> q1dot(1:12)"/1 -> Mux/1
  Selector/1 -> "q2dot(1:12) -> q1dot(1:12)"/1
  q2dot/1 -> Selector/1, Selector1/1
  Selector1/1 -> Demux/1
  Demux/1 -> Wheel revs FL/1
  Demux/2 -> Wheel revs FR/1
  Demux/3 -> Wheel revs RL/1
  Demux/4 -> Wheel revs RR/1
  Wheel revs reset/1 -> Demux1/1
  Demux1/1 -> Wheel revs FL/2
  Demux1/2 -> Wheel revs FR/2
  Demux1/3 -> Wheel revs RL/2
  Demux1/4 -> Wheel revs RR/2
  Wheel revs FL/1 -> Mux/2
  Wheel revs FR/1 -> Mux/3
  Wheel revs RL/1 -> Mux/4
  Wheel revs RR/1 -> Mux/5

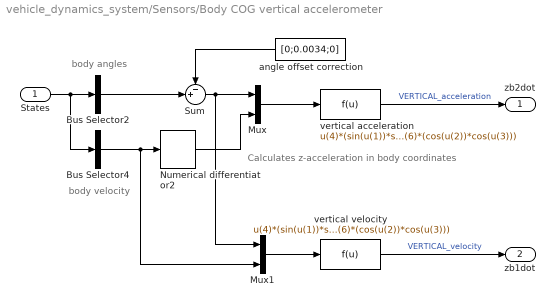
== system vehicle_dynamics_system/Sensors/Body COG vertical accelerometer ==
  note: Calculates z-acceleration
      | in body coordinates
  note: body velocity
  note: body angles
  States : Inport
  Bus Selector2 : BusSelector  OutputSignals=PSI_eulerangle,THETA_eulerangle,PHI_eulerangle  OutputAsBus=on
  Bus Selector4 : BusSelector  OutputSignals=X1dot_velocity,Y1dot_velocity,Z1dot_velocity  OutputAsBus=on
  Mux : Mux  Inputs=2
  Mux1 : Mux  Inputs=2
  Numerical differentiator2 : vehicle_dynamics_lib/Helper blocks/Numerical differentiator  SystemSampleTime=-1  Ts=0.01
  Sum : Sum  Inputs=-+|
  angle offset correction : Constant  Value=[0;0.0034;0]
  vertical acceleration : Fcn  Expr=u(4)*(sin(u(1))*sin(u(3))+cos(u(1))*sin(u(2))*cos(u(3)))+u(5)*(-cos(u(1))*sin(u(3))+sin(u(1))*sin(u(2))*cos(u(3)))+u(6)*(cos(u(2))*cos(u(3)))
  vertical velocity : Fcn  Expr=u(4)*(sin(u(1))*sin(u(3))+cos(u(1))*sin(u(2))*cos(u(3)))+u(5)*(-cos(u(1))*sin(u(3))+sin(u(1))*sin(u(2))*cos(u(3)))+u(6)*(cos(u(2))*cos(u(3)))
  zb2dot : Outport
  zb1dot : Outport  Port=2
  wires:
  Mux/1 -> vertical acceleration/1
  Numerical differentiator2/1 -> Mux/2
  Bus Selector4/1 -> Numerical differentiator2/1, Mux1/2
  States/1 -> Bus Selector2/1, Bus Selector4/1
  vertical acceleration/1 -> zb2dot/1  "VERTICAL_acceleration"
  Sum/1 -> Mux/1, Mux1/1
  Bus Selector2/1 -> Sum/2
  angle offset correction/1 -> Sum/1
  Mux1/1 -> vertical velocity/1
  vertical velocity/1 -> zb1dot/1  "VERTICAL_velocity"

== system vehicle_dynamics_system/Sensors/Body angular accelerometers ==
  States : Inport
  Bus Selector3 : BusSelector  OutputSignals=THETA1dot_angularvelocity,PHI1dot_angularvelocity
  Numerical differentiator : vehicle_dynamics_lib/Helper blocks/Numerical differentiator  SystemSampleTime=-1  Ts=0.01
  Numerical differentiator1 : vehicle_dynamics_lib/Helper blocks/Numerical differentiator  SystemSampleTime=-1  Ts=0.01
  theta2dot : Outport
  phi2dot : Outport  Port=2
  theta1dot : Outport  Port=3
  phi1dot : Outport  Port=4
  wires:
  Bus Selector3/1 -> Numerical differentiator/1, theta1dot/1  "<THETA1dot_angularvelocity>"
  Bus Selector3/2 -> Numerical differentiator1/1, phi1dot/1  "<PHI1dot_angularvelocity>"
  States/1 -> Bus Selector3/1
  Numerical differentiator/1 -> theta2dot/1  "THETA2dot_angularacceleration"
  Numerical differentiator1/1 -> phi2dot/1  "PHI2dot_angularacceleration"

== system vehicle_dynamics_system/Simple combustion engine/Rev limiter ==
  note: Limit revs of engine by hysteresis
  Revs : Inport
  Th in : Inport  Port=2
  Product : Product  RndMeth=Zero
  Relay : Relay  OnSwitchValue=Engine.MaxRPM  OffSwitchValue=Engine.MaxRPM-Engine.RevLimiterHysteresis  OnOutputValue=0  OffOutputValue=1
  Th out : Outport
  wires:
  Relay/1 -> Product/1
  Revs/1 -> Relay/1
  Th in/1 -> Product/2
  Product/1 -> Th out/1

== system vehicle_dynamics_system/Chassis/Air resistance forces & downforce calculation/Air resistance ==
  note: F_{Drag} = -1/2 \cdot \rho \cdot A \cdot C_w \cdot sign(v_x) \cdot v_x^2
  note: The output force is also divided by 2 because it is assumed that the air
      | drag force is equally applied to the front and rear point of attack.
  v_x : Inport
  Gain : Gain  Gain=-.25
  Math Function : Math  Operator=square  SaturateOnIntegerOverflow=on
  Product : Product  RndMeth=Zero
  Sign : Signum
  air density : Gain  Gain=rho
  drag coefficient : Gain  Gain=Cw
  reference area : Gain  Gain=A
  F_Drag : Outport
  wires:
  Math Function/1 -> air density/1
  air density/1 -> reference area/1
  reference area/1 -> drag coefficient/1
  drag coefficient/1 -> Gain/1
  v_x/1 -> Math Function/1, Sign/1
  Gain/1 -> Product/1
  Product/1 -> F_Drag/1
  Sign/1 -> Product/2

== system vehicle_dynamics_system/Chassis/Air resistance forces & downforce calculation/Downforce ==
  note: F_{Downforce} = -1/2 \cdot \rho \cdot K_s \cdot v_x^2
  v_x : Inport
  Gain : Gain  Gain=-.5
  Math Function : Math  Operator=square  SaturateOnIntegerOverflow=on
  air density : Gain  Gain=rho
  wing coefficient front : Gain  Gain=Ksfront
  wing coefficient rear : Gain  Gain=Ksrear
  F_DownforceFront : Outport
  F_DownforceRear : Outport  Port=2
  wires:
  v_x/1 -> Math Function/1
  Math Function/1 -> air density/1
  air density/1 -> Gain/1
  Gain/1 -> wing coefficient front/1, wing coefficient rear/1
  wing coefficient front/1 -> F_DownforceFront/1
  wing coefficient rear/1 -> F_DownforceRear/1
